simulink library "MEKF_ValidityTest_Lib2018"  (R2018b)
settings: Solver=VariableStepAuto  StartTime=0.0  StopTime=10.0  RelTol=1e-3
values from neighbouring files (symbols this model uses):
  Beta_init = Beta    [MEKF_ScriptandSimulink_Test.m]
  del_t = tspan(2)-tspan(1)    [MEKF_ScriptandSimulink_Test.m]
  P_sq_init = P_sq    [MEKF_ScriptandSimulink_Test.m]
  q = [q(:,2),q(:,3),q(:,4),q(:,1)]    [MEKF_ScriptandSimulink_Test.m]
  Q_sq = chol((gamma*Q_k*gamma'),'lower')    [MEKF_ScriptandSimulink_Test.m]
  qe_init = qe    [MEKF_ScriptandSimulink_Test.m]
  R_sq = chol(R,'lower')    [MEKF_ScriptandSimulink_Test.m]
libraries: MEKF_LibraryR2018b x13, aerolibutil x12, dspmtrx3 x7, sharedutil x6, $bdroot x2
(part 2 of 2)

== system MEKF_ValidityTest_Lib2018/MEKF with Validity Check/If All Sensors Valid/Kalman Gain ==
  P_sq : Inport
  q_est : Inport  Port=2
  SunVector_Inertial : Inport  Port=3
  "Mag_vec " : Inport  Port=4
  Constant : Constant  Value=R_sq  VectorParams1D=off
  Create H matrix : Subsystem
  Demux : Demux
  Divide : Product  Inputs=/  Multiplication=Matrix(*)
  MATLAB Function2 : MATLAB Function  TreatAsAtomicUnit=on
  Makes Xi(q) Matrix : Subsystem
  Matrix Concatenate : Concatenate  Mode=Multidimensional array
  Matrix Multiply1 : Product  Multiplication=Matrix(*)
  Mux : Mux
  Quaternion Rotation : aerolibutil/Quaternion Rotation
  Quaternion Rotation1 : aerolibutil/Quaternion Rotation
  P_square root plus : Outport
  Xi(q) : Outport  Port=2
  est_measurement : Outport  Port=3
  Kalman Gain K : Outport  Port=4
  wires:
  Divide/1 -> Matrix Multiply1/2
  MATLAB Function2/1(W) -> Matrix Multiply1/1
  Create H matrix/1(H) -> MATLAB Function2/3(H)  "Sensitivity Matrix"
  MATLAB Function2/2(sq_Bk) -> Divide/1
  P_sq/1 -> MATLAB Function2/2("P_sq ")
  Matrix Multiply1/1 -> Kalman Gain K/1  "Kalman Gain K"
  SunVector_Inertial/1 -> Quaternion Rotation/2
  Constant/1 -> MATLAB Function2/1(R_sq)
  MATLAB Function2/3(P_sq) -> P_square root plus/1  "P_square root plus"
  Demux/1 -> Mux/2
  Demux/2 -> Mux/3
  Demux/3 -> Mux/4
  Demux/4 -> Mux/1
  Makes Xi(q) Matrix/1(Xi(q)) -> Xi(q)/1
  q_est/1 -> [q_est]
  [q_est] -> Demux/1
  [q_est] -> Makes Xi(q) Matrix/1(qest)
  Quaternion Rotation/1 -> [rb_hat]  "product A(q)*R_i"
  [rb_hat] -> Create H matrix/1(rb_hat)
  "Mag_vec "/1 -> Quaternion Rotation1/2
  Quaternion Rotation1/1 -> [bhat]  "product A(q)*B_i"
  Mux/1 -> [qmix]
  [qmix] -> Quaternion Rotation1/1
  [qmix] -> Quaternion Rotation/1
  [bhat] -> Create H matrix/2(bb_hat)
  [rb_hat] -> Matrix Concatenate/1
  [bhat] -> Matrix Concatenate/2
  Matrix Concatenate/1 -> est_measurement/1

== system MEKF_ValidityTest_Lib2018/MEKF with Validity Check/If All Sensors Valid/MEASUREMENT UPDATE TO q AND COVARIANCE2 ==
  Xi_q : Inport
  r_est : Inport  Port=2
  Kalman Gain : Inport  Port=3
  q_est minus : Inport  Port=4
  Beta_est : Inport  Port=5
  Rb : Inport  Port=6
  Create Measurement Residual : Sum  Inputs=+-
  Demux : Demux  Outputs=2
  Normalize_q : Subsystem
  Product : Product  Inputs=**  Multiplication=Matrix(*)
  Product1 : Product  Multiplication=Matrix(*)
  Sum : Sum  Inputs=|++
  "Updating Beta Bias " : Sum  Inputs=|++
  gain1 : Gain  Gain=0.5
  Measurement updated q estimate : Outport
  Beta Updated : Outport  Port=2
  wires:
  Demux/1 -> Product/2  "Delta Alpha"
  gain1/1 -> Product/1  "0.5*Xi_q"
  Demux/2 -> "Updating Beta Bias "/1  "Delta Beta"
  Product/1 -> Sum/1
  Product1/1 -> Demux/1  "del_x"
  r_est/1 -> Create Measurement Residual/2
  Create Measurement Residual/1 -> Product1/2  "Measurement Residual"
  "Updating Beta Bias "/1 -> Beta Updated/1  "Beta Updated"
  Beta_est/1 -> "Updating Beta Bias "/2  "Beta_estimated"
  q_est minus/1 -> Sum/2
  Kalman Gain/1 -> Product1/1
  Rb/1 -> Create Measurement Residual/1
  Xi_q/1 -> gain1/1  "quaternion Propagation Matrix"
  Sum/1 -> Normalize_q/1(Estimated Quaternion)  "Estimated Quaternion"
  Normalize_q/1(q_normalized) -> Measurement updated q estimate/1

== system MEKF_ValidityTest_Lib2018/MEKF with Validity Check/If All Sensors Valid/TIME PROPAGATION of Q_EST, COVARIANCE ==
  P_square root plus : Inport
  qe : Inport  Port=2
  Updated bias : Inport  Port=3
  omega_meas : Inport  Port=4
  Constant{,1..3} (4 alike) : Constant  Value=del_t
  Constant11 : Constant  Value=0.5
  Constant13 : Constant  Value=Q_sq  VectorParams1D=off
  Gain : Gain  Gain=0.5
  MATLAB Function : MATLAB Function  TreatAsAtomicUnit=on
  MATLAB Function1 : MATLAB Function  TreatAsAtomicUnit=on
  MATLAB Function10 : MATLAB Function  TreatAsAtomicUnit=on
  MATLAB Function11 : MATLAB Function  TreatAsAtomicUnit=on
  MATLAB Function7 : MATLAB Function  TreatAsAtomicUnit=on
  MATLAB Function8 : MATLAB Function  TreatAsAtomicUnit=on
  MATLAB Function9 : MATLAB Function  TreatAsAtomicUnit=on
  Product : Product  Multiplication=Matrix(*)
  Psi : Subsystem
  cos_omega : Subsystem
  SqR P(k+1) : Outport
  qest(k+1) : Outport  Port=2
  Angular Velo Est : Outport  Port=3
  wires:
  Constant3/1 -> MATLAB Function8/4(del_t)
  MATLAB Function7/1(Psi_cross) -> MATLAB Function8/1(Psi_x)
  MATLAB Function11/1(P_sq) -> SqR P(k+1)/1  "C gets QR decomped to propagate sqrt(P)"
  MATLAB Function8/1(Omega_omega) -> Product/1  "q propagation matrix (nothing to do with angular velo)"
  MATLAB Function9/1(omega_cross_matrix) -> MATLAB Function10/4(omega_x)
  MATLAB Function10/1(State_Trans_matrix) -> MATLAB Function11/1(Phi_discrete)  "State Transition matrix to proagate P"
  Product/1 -> qest(k+1)/1  "Time Propagated q"
  Constant13/1 -> MATLAB Function11/2(Q_sq)  "process noise chol decomped covariance matrix"
  omega_meas/1 -> MATLAB Function1/2(mu)
  Updated bias/1 -> MATLAB Function1/1(nu)
  MATLAB Function/1(om_mag) -> [om_mag]  "om_mag"
  [om_mag] -> MATLAB Function10/3(om_mag)
  [om_mag] -> MATLAB Function8/3(om_mag)
  Constant1/1 -> MATLAB Function10/1(del_t)
  P_square root plus/1 -> [P_sq_plus]
  [P_sq_plus] -> MATLAB Function11/3("P_sq ")
  [omega_estj] -> MATLAB Function9/1(omega)
  [nonmergew] -> Angular Velo Est/1
  qe/1 -> [qe]
  [qe] -> Product/2
  [om_mag] -> cos_omega/1(In1)
  Constant/1 -> cos_omega/2(In2)
  [om_mag] -> cos_omega/3(In3)
  cos_omega/1(cos_omega) -> MATLAB Function10/2(cos_omega)  "cos_omega"
  Psi/1(Psi) -> MATLAB Function8/2(Psi), MATLAB Function7/1(Psi)  "Psi Matrix"
  Constant2/1 -> Psi/1(In1)
  Constant11/1 -> Psi/2(In2)
  [omega_estj] -> Psi/5(In4)
  [om_mag] -> Psi/3(In3), Psi/4(In5)
  MATLAB Function1/2(om_estbranch) -> Gain/1  "omega est"
  Gain/1 -> [omega_estj], MATLAB Function/1(omega_est)
  MATLAB Function1/1(om_est) -> [nonmergew]  "om_mag"

== system MEKF_ValidityTest_Lib2018/MEKF with Validity Check/If Gyros Valid, Sun or Mag Sensor Invlaid/Subsystem ==
  P_sq : Inport
  q_est1 : Inport  Port=2
  SunVector_Inertial : Inport  Port=3
  "Mag_vec " : Inport  Port=4
  Constant : Constant  Value=R_sq*100000000  VectorParams1D=off
  Create H matrix : MEKF_LibraryR2018b/Multiplicative Extended Kalman Filter/Kalman Gain/Create H matrix  SystemSampleTime=-1
  Demux : Demux
  Divide : Product  Inputs=/  Multiplication=Matrix(*)
  MATLAB Function2 : MEKF_LibraryR2018b/Multiplicative Extended Kalman Filter/Kalman Gain/MATLAB Function2  SystemSampleTime=-1
  Makes Xi(q) Matrix : MEKF_LibraryR2018b/Multiplicative Extended Kalman Filter/Kalman Gain/Makes Xi(q) Matrix  SystemSampleTime=-1
  Matrix Concatenate : Concatenate  Mode=Multidimensional array
  Matrix Multiply1 : Product  Multiplication=Matrix(*)
  Mux2 : Mux
  Quaternion Rotation2 : aerolibutil/Quaternion Rotation
  Quaternion Rotation3 : aerolibutil/Quaternion Rotation
  Xi(q) : Outport
  Kalman Gain K : Outport  Port=2
  P_square root plus : Outport  Port=3
  est_measurement : Outport  Port=4
  wires:
  Mux2/1 -> [qmix]
  q_est1/1 -> [q_est]
  P_sq/1 -> MATLAB Function2/2
  [q_est] -> Demux/1
  Demux/2 -> Mux2/3
  [q_est] -> Makes Xi(q) Matrix/1
  "Mag_vec "/1 -> Quaternion Rotation3/2
  Matrix Concatenate/1 -> est_measurement/1
  [bhat] -> Create H matrix/2
  Demux/1 -> Mux2/2
  [rb_hat] -> Matrix Concatenate/1
  Demux/4 -> Mux2/1
  [bhat] -> Matrix Concatenate/2
  [rb_hat] -> Create H matrix/1
  Quaternion Rotation2/1 -> [rb_hat]  "product A(q)*R_i"
  Quaternion Rotation3/1 -> [bhat]  "product A(q)*B_i"
  [qmix] -> Quaternion Rotation3/1
  Divide/1 -> Matrix Multiply1/2
  SunVector_Inertial/1 -> Quaternion Rotation2/2
  [qmix] -> Quaternion Rotation2/1
  Demux/3 -> Mux2/4
  Makes Xi(q) Matrix/1 -> Xi(q)/1
  MATLAB Function2/2 -> Divide/1
  Matrix Multiply1/1 -> Kalman Gain K/1  "Kalman Gain K"
  MATLAB Function2/3 -> P_square root plus/1  "P_square root plus"
  Create H matrix/1 -> MATLAB Function2/3  "Sensitivity Matrix"
  MATLAB Function2/1 -> Matrix Multiply1/1
  Constant/1 -> MATLAB Function2/1

== system MEKF_ValidityTest_Lib2018/MEKF with Validity Check/If Gyros Valid, Sun or Mag Sensor Invlaid/Subsystem1 ==
  Xi_q : Inport
  r_est : Inport  Port=2
  Kalman Gain : Inport  Port=3
  q_est minus : Inport  Port=4
  Beta_est : Inport  Port=5
  Rb : Inport  Port=6
  Create Measurement Residual : Sum  Inputs=+-
  Demux : Demux  Outputs=2
  Normalize_q : MEKF_LibraryR2018b/Multiplicative Extended Kalman Filter/MEASUREMENT UPDATE TO q AND COVARIANCE2/Normalize_q  SystemSampleTime=-1
  Product : Product  Inputs=**  Multiplication=Matrix(*)
  Product1 : Product  Multiplication=Matrix(*)
  Sum : Sum  Inputs=|++
  "Updating Beta Bias " : Sum  Inputs=|++
  gain1 : Gain  Gain=0.5
  Measurement updated q estimate : Outport
  Beta Updated : Outport  Port=2
  wires:
  Demux/2 -> "Updating Beta Bias "/1  "Delta Beta"
  Xi_q/1 -> gain1/1
  "Updating Beta Bias "/1 -> Beta Updated/1  "Beta Updated"
  Kalman Gain/1 -> Product1/1
  Create Measurement Residual/1 -> Product1/2  "Measurement Residual"
  Rb/1 -> Create Measurement Residual/1
  Demux/1 -> Product/2  "Delta Alpha"
  r_est/1 -> Create Measurement Residual/2
  Sum/1 -> Normalize_q/1  "Estimated Quaternion"
  Beta_est/1 -> "Updating Beta Bias "/2
  q_est minus/1 -> Sum/2
  Normalize_q/1 -> Measurement updated q estimate/1
  gain1/1 -> Product/1  "0.5*Xi_q"
  Product/1 -> Sum/1
  Product1/1 -> Demux/1  "del_x"

== system MEKF_ValidityTest_Lib2018/MEKF with Validity Check/If Gyros Valid, Sun or Mag Sensor Invlaid/Subsystem2 ==
  Square Root Covariane at next Time step becomes sqrt Pk minus : Inport
  Matrix Multiply : Product  Multiplication=Matrix(*)
  Transpose : Math  Operator=transpose  SaturateOnIntegerOverflow=on
  Out1 : Outport
  wires:
  Matrix Multiply/1 -> Out1/1
  Transpose/1 -> Matrix Multiply/2
  Square Root Covariane at next Time step becomes sqrt Pk minus/1 -> Transpose/1, Matrix Multiply/1

== system MEKF_ValidityTest_Lib2018/MEKF with Validity Check/If Gyros Valid, Sun or Mag Sensor Invlaid/Subsystem3 ==
  P_square root plus : Inport
  qe : Inport  Port=2
  Updated bias : Inport  Port=3
  omega_meas : Inport  Port=4
  Constant10 : Constant  Value=del_t
  Constant11 : Constant  Value=0.5
  Constant13 : Constant  Value=Q_sq  VectorParams1D=off
  MATLAB Function : MEKF_LibraryR2018b/Multiplicative Extended Kalman Filter/TIME PROPAGATION of Q_EST, COVARIANCE/MATLAB Function  SystemSampleTime=-1
  MATLAB Function10 : MEKF_LibraryR2018b/Multiplicative Extended Kalman Filter/TIME PROPAGATION of Q_EST, COVARIANCE/MATLAB Function10  SystemSampleTime=-1
  MATLAB Function11 : MEKF_LibraryR2018b/Multiplicative Extended Kalman Filter/TIME PROPAGATION of Q_EST, COVARIANCE/MATLAB Function11  SystemSampleTime=-1
  MATLAB Function7 : MEKF_LibraryR2018b/Multiplicative Extended Kalman Filter/TIME PROPAGATION of Q_EST, COVARIANCE/MATLAB Function7  SystemSampleTime=-1
  MATLAB Function8 : MEKF_LibraryR2018b/Multiplicative Extended Kalman Filter/TIME PROPAGATION of Q_EST, COVARIANCE/MATLAB Function8  SystemSampleTime=-1
  MATLAB Function9 : MEKF_LibraryR2018b/Multiplicative Extended Kalman Filter/TIME PROPAGATION of Q_EST, COVARIANCE/MATLAB Function9  SystemSampleTime=-1
  Product : Product  Multiplication=Matrix(*)
  Psi : MEKF_LibraryR2018b/Multiplicative Extended Kalman Filter/TIME PROPAGATION of Q_EST, COVARIANCE/Psi  SystemSampleTime=-1
  cos_omega : MEKF_LibraryR2018b/Multiplicative Extended Kalman Filter/TIME PROPAGATION of Q_EST, COVARIANCE/cos_omega  SystemSampleTime=-1
  subtract bias from omega meas : Sum  Inputs=|-+
  SqR P(k+1) : Outport
  qest(k+1) : Outport  Port=2
  Angular Velo Est : Outport  Port=3
  wires:
  MATLAB Function/1 -> [om_mag]  "om_mag"
  Psi/1 -> MATLAB Function8/2, MATLAB Function7/1  "Psi Matrix"
  [om_mag] -> Psi/3, Psi/4
  Constant11/1 -> Psi/2
  [qe] -> Product/2
  [del_t] -> Psi/1
  [omega_est] -> Angular Velo Est/1
  [del_t] -> MATLAB Function10/1
  [om_mag] -> MATLAB Function8/3
  MATLAB Function8/1 -> Product/1  "q propagation matrix (nothing to do with angular velo)"
  MATLAB Function10/1 -> MATLAB Function11/1  "State Transition matrix to proagate P"
  [omega_est] -> Psi/5
  [omega_est] -> MATLAB Function9/1
  [om_mag] -> MATLAB Function10/3
  [del_t] -> MATLAB Function8/4
  [del_t] -> cos_omega/2
  [om_mag] -> cos_omega/3
  MATLAB Function11/1 -> SqR P(k+1)/1  "C gets QR decomped to propagate sqrt(P)"
  [P_sq_plus] -> MATLAB Function11/3
  qe/1 -> [qe]
  P_square root plus/1 -> [P_sq_plus]
  MATLAB Function9/1 -> MATLAB Function10/4
  cos_omega/1 -> MATLAB Function10/2  "cos_omega"
  omega_meas/1 -> subtract bias from omega meas/2
  subtract bias from omega meas/1 -> MATLAB Function/1, [omega_est]  "omega est"
  Product/1 -> qest(k+1)/1  "Time Propagated q"
  Updated bias/1 -> subtract bias from omega meas/1
  Constant10/1 -> [del_t]  "del_t"
  MATLAB Function7/1 -> MATLAB Function8/1
  [om_mag] -> cos_omega/1
  Constant13/1 -> MATLAB Function11/2  "process noise chol decomped covariance matrix"

== system MEKF_ValidityTest_Lib2018/MEKF (All Sensors INVALID)/Kalman Gain/Create H matrix/3x3 0 matrix ==
  Create 3x3 Matrix : sharedutil/Create 3x3 Matrix  aMode=aMode
  Zero : Constant  Value=0  OutDataTypeStr=Inherit: Inherit via back propagation
  0 3x3 : Outport
  wires:
  Create 3x3 Matrix/1 -> 0 3x3/1
  Zero/1 -> Create 3x3 Matrix/4, Create 3x3 Matrix/3, Create 3x3 Matrix/2, Create 3x3 Matrix/5, Create 3x3 Matrix/1, Create 3x3 Matrix/6, Create 3x3 Matrix/7, Create 3x3 Matrix/8, Create 3x3 Matrix/9

== system MEKF_ValidityTest_Lib2018/MEKF (Sun, Mag:VALID Sensors Gyro: INVALID Sensor)/Kalman Gain/Create H matrix/3x3 0 matrix ==
  Create 3x3 Matrix : sharedutil/Create 3x3 Matrix  aMode=aMode
  Zero : Constant  Value=0  OutDataTypeStr=Inherit: Inherit via back propagation
  0 3x3 : Outport
  wires:
  Zero/1 -> Create 3x3 Matrix/9, Create 3x3 Matrix/8, Create 3x3 Matrix/7, Create 3x3 Matrix/6, Create 3x3 Matrix/1, Create 3x3 Matrix/5, Create 3x3 Matrix/2, Create 3x3 Matrix/3, Create 3x3 Matrix/4
  Create 3x3 Matrix/1 -> 0 3x3/1

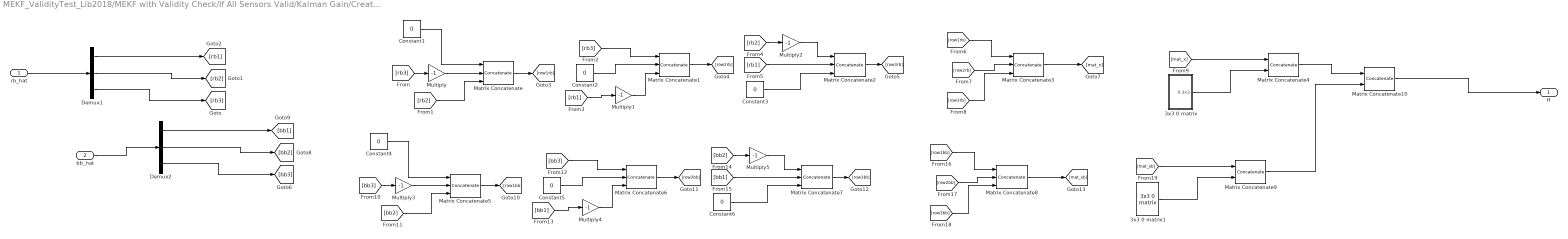
== system MEKF_ValidityTest_Lib2018/MEKF with Validity Check/If All Sensors Valid/Kalman Gain/Create H matrix ==
  rb_hat : Inport
  bb_hat : Inport  Port=2
  3x3 0 matrix : Subsystem
  3x3 0 matrix1 : MEKF_LibraryR2018b/Multiplicative Extended Kalman Filter/Kalman Gain/Create H matrix/3x3 0 matrix  SystemSampleTime=-1
  Constant{1..6} (6 alike) : Constant  Value=0
  Demux1 : Demux  Outputs=3
  Demux2 : Demux  Outputs=3
  Matrix Concatenate{,1..2,5..7} (6 alike) : Concatenate  NumInputs=3  Mode=Multidimensional array  ConcatenateDimension=2
  Matrix Concatenate10 : Concatenate  Mode=Multidimensional array
  Matrix Concatenate3 : Concatenate  NumInputs=3  Mode=Multidimensional array
  Matrix Concatenate4 : Concatenate  Mode=Multidimensional array  ConcatenateDimension=2
  Matrix Concatenate8 : Concatenate  NumInputs=3  Mode=Multidimensional array
  Matrix Concatenate9 : Concatenate  Mode=Multidimensional array  ConcatenateDimension=2
  Multiply{,1..5} (6 alike) : Gain  Gain=-1
  H : Outport
  wires:
  Matrix Concatenate1/1 -> [row2rb]
  Multiply/1 -> Matrix Concatenate/2
  [mat_x] -> Matrix Concatenate4/1
  Demux1/2 -> [rb2]
  Multiply2/1 -> Matrix Concatenate2/1
  [row3rb] -> Matrix Concatenate3/3
  Matrix Concatenate/1 -> [row1rb]
  Matrix Concatenate2/1 -> [row3rb]
  [rb1] -> Multiply1/1
  [rb3] -> Multiply/1
  Multiply1/1 -> Matrix Concatenate1/3
  Constant3/1 -> Matrix Concatenate2/3
  3x3 0 matrix/1(0 3x3) -> Matrix Concatenate4/2
  [rb2] -> Multiply2/1
  [rb2] -> Matrix Concatenate/3
  [rb3] -> Matrix Concatenate1/1
  [row2rb] -> Matrix Concatenate3/2
  Constant1/1 -> Matrix Concatenate/1
  [row1rb] -> Matrix Concatenate3/1
  Demux1/1 -> [rb1]
  Matrix Concatenate3/1 -> [mat_x]
  Constant2/1 -> Matrix Concatenate1/2
  [rb1] -> Matrix Concatenate2/2
  Demux1/3 -> [rb3]
  rb_hat/1 -> Demux1/1
  Demux2/3 -> [bb3]
  bb_hat/1 -> Demux2/1
  Demux2/1 -> [bb1]
  Demux2/2 -> [bb2]
  Multiply5/1 -> Matrix Concatenate7/1
  [bb1] -> Matrix Concatenate7/2
  Constant4/1 -> Matrix Concatenate5/1
  Multiply3/1 -> Matrix Concatenate5/2
  Constant5/1 -> Matrix Concatenate6/2
  Multiply4/1 -> Matrix Concatenate6/3
  Matrix Concatenate5/1 -> [row1bb]
  [bb1] -> Multiply4/1
  Matrix Concatenate7/1 -> [row3bb]
  Constant6/1 -> Matrix Concatenate7/3
  [bb2] -> Matrix Concatenate5/3
  [bb3] -> Multiply3/1
  [bb3] -> Matrix Concatenate6/1
  [bb2] -> Multiply5/1
  Matrix Concatenate6/1 -> [row2bb]
  [row1bb] -> Matrix Concatenate8/1
  Matrix Concatenate8/1 -> [mat_xb]
  [row2bb] -> Matrix Concatenate8/2
  [row3bb] -> Matrix Concatenate8/3
  3x3 0 matrix1/1 -> Matrix Concatenate9/2
  Matrix Concatenate9/1 -> Matrix Concatenate10/2
  [mat_xb] -> Matrix Concatenate9/1
  Matrix Concatenate4/1 -> Matrix Concatenate10/1
  Matrix Concatenate10/1 -> H/1

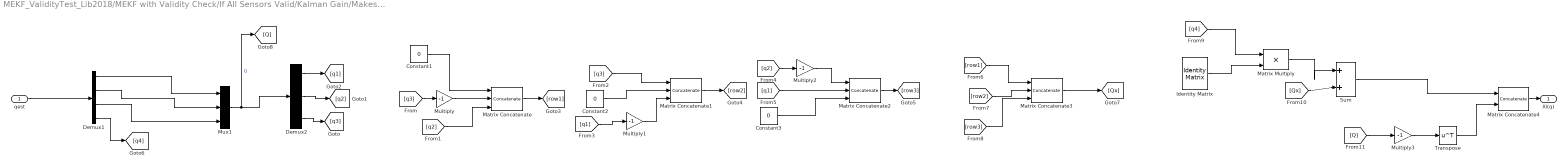
== system MEKF_ValidityTest_Lib2018/MEKF with Validity Check/If All Sensors Valid/Kalman Gain/Makes Xi(q) Matrix ==
  qest : Inport
  Constant1 : Constant  Value=0
  Constant2 : Constant  Value=0
  Constant3 : Constant  Value=0
  Demux1 : Demux
  Demux2 : Demux  Outputs=3
  Identity Matrix : dspmtrx3/Identity Matrix  Inherit=off  N=3  Ts=1  dataType=double  isSigned=on  wordLen=16  udDataType=sfix(16)  fracBitsMode=Best precision  numFracBits=15  OutDataTypeStr=double  LastOutDataTypeStr=double
      settings: SourceProductName=DSP System Toolbox
  Matrix Concatenate : Concatenate  NumInputs=3  Mode=Multidimensional array  ConcatenateDimension=2
  Matrix Concatenate1 : Concatenate  NumInputs=3  Mode=Multidimensional array  ConcatenateDimension=2
  Matrix Concatenate2 : Concatenate  NumInputs=3  Mode=Multidimensional array  ConcatenateDimension=2
  Matrix Concatenate3 : Concatenate  NumInputs=3  Mode=Multidimensional array
  Matrix Concatenate4 : Concatenate  Mode=Multidimensional array
  Matrix Multiply : Product  Inputs=**
  Multiply{,1..3} (4 alike) : Gain  Gain=-1
  Mux1 : Mux  Inputs=3
  Sum : Sum  Inputs=|++
  Transpose : Math  Operator=transpose  SaturateOnIntegerOverflow=on
  Xi(q) : Outport
  wires:
  Multiply2/1 -> Matrix Concatenate2/1
  [q1] -> Matrix Concatenate2/2
  Matrix Multiply/1 -> Sum/1
  Matrix Concatenate1/1 -> [row2]
  Constant1/1 -> Matrix Concatenate/1
  Matrix Concatenate3/1 -> [Qx]
  [q2] -> Matrix Concatenate/3
  Mux1/1 -> Demux2/1, [Q]  "Q"
  Constant2/1 -> Matrix Concatenate1/2
  Demux1/2 -> Mux1/2
  [row3] -> Matrix Concatenate3/3
  qest/1 -> Demux1/1
  Multiply3/1 -> Transpose/1
  [q4] -> Matrix Multiply/1
  [q3] -> Matrix Concatenate1/1
  Demux2/2 -> [q2]
  Sum/1 -> Matrix Concatenate4/1
  [q2] -> Multiply2/1
  Demux1/4 -> [q4]
  [row2] -> Matrix Concatenate3/2
  Demux1/1 -> Mux1/1
  Demux1/3 -> Mux1/3
  Matrix Concatenate2/1 -> [row3]
  [Qx] -> Sum/2
  Multiply/1 -> Matrix Concatenate/2
  [row1] -> Matrix Concatenate3/1
  [Q] -> Multiply3/1
  Demux2/1 -> [q1]
  Transpose/1 -> Matrix Concatenate4/2
  Identity Matrix/1 -> Matrix Multiply/2
  [q3] -> Multiply/1
  Matrix Concatenate/1 -> [row1]
  Demux2/3 -> [q3]
  Constant3/1 -> Matrix Concatenate2/3
  [q1] -> Multiply1/1
  Multiply1/1 -> Matrix Concatenate1/3
  Matrix Concatenate4/1 -> Xi(q)/1

== system MEKF_ValidityTest_Lib2018/MEKF with Validity Check/If All Sensors Valid/MEASUREMENT UPDATE TO q AND COVARIANCE2/Normalize_q ==
  note: Rearrange_Quat
  note: Rearrange_Quat_back
  Estimated Quaternion : Inport
  Demux : Demux
  Demux1 : Demux
  Mux : Mux
  Mux1 : Mux
  Quaternion Normalize : sharedutil/Quaternion Normalize  aMode=aMode
      settings: SourceProductName=Aerospace Blockset  SourceProductBaseCode=AE
  q_normalized : Outport
  wires:
  Mux1/1 -> Quaternion Normalize/1
  Demux1/4 -> Mux1/1
  Demux/4 -> Mux/3
  Demux/3 -> Mux/2
  Demux/2 -> Mux/1
  Demux1/3 -> Mux1/4
  Mux/1 -> q_normalized/1
  Demux1/1 -> Mux1/2
  Demux1/2 -> Mux1/3
  Demux/1 -> Mux/4
  Quaternion Normalize/1 -> Demux/1  "Measurement updated q estimate"
  Estimated Quaternion/1 -> Demux1/1

== system MEKF_ValidityTest_Lib2018/MEKF with Validity Check/If All Sensors Valid/TIME PROPAGATION of Q_EST, COVARIANCE/Psi ==
  In1 : Inport
  In2 : Inport  Port=2
  In3 : Inport  Port=3
  In5 : Inport  Port=4
  In4 : Inport  Port=5
  Divide : Product  Inputs=***
  Divide1 : Product  Inputs=**/
  Sin : Trigonometry
  Psi : Outport
  wires:
  In1/1 -> Divide/1
  Divide/1 -> Sin/1  "om_mag times0.5*del_t"
  In5/1 -> Divide1/3
  In4/1 -> Divide1/2
  Divide1/1 -> Psi/1  "Psi"
  In3/1 -> Divide/3
  Sin/1 -> Divide1/1  "sin(om_mag*0.5*del_t)"
  In2/1 -> Divide/2

== system MEKF_ValidityTest_Lib2018/MEKF with Validity Check/If All Sensors Valid/TIME PROPAGATION of Q_EST, COVARIANCE/cos_omega ==
  In1 : Inport
  In2 : Inport  Port=2
  In3 : Inport  Port=3
  Constant12 : Constant
  Cos : Trigonometry  Operator=cos
  Divide2 : Product  Inputs=**
  Divide3 : Product  Inputs=*/
  Square : Math  Operator=square  SaturateOnIntegerOverflow=on
  Sum3 : Sum  Inputs=|+-
  cos_omega : Outport
  wires:
  Divide2/1 -> Cos/1
  In3/1 -> Square/1
  Divide3/1 -> cos_omega/1  "cos_omega"
  Constant12/1 -> Sum3/1
  Square/1 -> Divide3/2  "omega mag squared"
  In1/1 -> Divide2/1
  Cos/1 -> Sum3/2
  In2/1 -> Divide2/2
  Sum3/1 -> Divide3/1  "(1-cos(om_mag*del_t))"

== system MEKF_ValidityTest_Lib2018/MEKF with Validity Check/If All Sensors Valid/Kalman Gain/Create H matrix/3x3 0 matrix ==
  Create 3x3 Matrix : sharedutil/Create 3x3 Matrix  aMode=aMode
  Zero : Constant  Value=0  OutDataTypeStr=Inherit: Inherit via back propagation
  0 3x3 : Outport
  wires:
  Zero/1 -> Create 3x3 Matrix/9, Create 3x3 Matrix/8, Create 3x3 Matrix/7, Create 3x3 Matrix/6, Create 3x3 Matrix/1, Create 3x3 Matrix/5, Create 3x3 Matrix/2, Create 3x3 Matrix/3, Create 3x3 Matrix/4
  Create 3x3 Matrix/1 -> 0 3x3/1

== matlab function MEKF_ValidityTest_Lib2018/MEKF with Validity Check/If All Sensors Valid/Kalman Gain/MATLAB Function2 ==
  data: R_sq input; W output; P_sq input; H input; sq_Bk output; P_sq output
function [W,sq_Bk,P_sq] = fcnAQR(R_sq,P_sq,H)
%#codegen
[nr,mr] = size(R_sq);
[np,mp] = size(P_sq);
A_QR = [R_sq',zeros(nr,np);(P_sq')*H', P_sq'];

[TA,UA] = qr(A_QR);
        P_sq = UA(7:12,7:12)'; %Updated P_sq
        W = UA(1:6,7:12)';
%        
        sq_Bk = UA(1:6,1:6)';

== matlab function MEKF_ValidityTest_Lib2018/MEKF with Validity Check/If All Sensors Valid/TIME PROPAGATION of Q_EST, COVARIANCE/MATLAB Function1 ==
  data: nu input; om_est output; mu input; om_estbranch output
function [om_est,om_estbranch] = om2_est(nu,mu)

om_est = mu-nu;
om_estbranch =2*( mu-nu);

== matlab function MEKF_ValidityTest_Lib2018/MEKF with Validity Check/If All Sensors Valid/TIME PROPAGATION of Q_EST, COVARIANCE/MATLAB Function7 ==
  data: Psi input; Psi_cross output
function Psi_cross = Psi_cross_matrix(Psi)
%#codegen

Psi_cross = [0 -Psi(3) Psi(2);Psi(3) 0 -Psi(1);-Psi(2) Psi(1) 0];

== matlab function MEKF_ValidityTest_Lib2018/MEKF with Validity Check/If All Sensors Valid/TIME PROPAGATION of Q_EST, COVARIANCE/MATLAB Function8 ==
  data: Psi_x input; Psi input; om_mag input; del_t input; Omega_omega output
function Omega_omega = omega_omega_matrix(Psi_x,Psi,om_mag,del_t)
%#codegen

 Omega_omega = [(cos(0.5*om_mag*del_t)*eye(3) - Psi_x), Psi; -Psi', cos(0.5*om_mag*del_t)];

== matlab function MEKF_ValidityTest_Lib2018/MEKF with Validity Check/If All Sensors Valid/TIME PROPAGATION of Q_EST, COVARIANCE/MATLAB Function9 ==
  data: omega input; omega_cross_matrix output
function omega_cross_matrix = makes_omega_cross_matrix(omega)

omega_cross_matrix = [0 -omega(3) omega(2);omega(3) 0 -omega(1);-omega(2) omega(1) 0];

== matlab function MEKF_ValidityTest_Lib2018/MEKF with Validity Check/If All Sensors Valid/TIME PROPAGATION of Q_EST, COVARIANCE/MATLAB Function10 ==
  data: del_t input; cos_omega input; om_mag input; omega_x input; State_Trans_matrix output
function State_Trans_matrix = Phi_disc(del_t,cos_omega,om_mag,omega_x)
%#codegen

State_Trans_matrix = [(eye(3)-omega_x*sin(om_mag*del_t)/om_mag + (omega_x^2)*cos_omega),omega_x*cos_omega-eye(3)*del_t-omega_x^2*(om_mag*del_t-sin(om_mag*del_t))/om_mag^3;
            zeros(3,3),eye(3)];

== matlab function MEKF_ValidityTest_Lib2018/MEKF with Validity Check/If All Sensors Valid/TIME PROPAGATION of Q_EST, COVARIANCE/MATLAB Function11 ==
  data: Phi_discrete input; P_sq output; Q_sq input; P_sq input
function P_sq  = Cqr(Phi_discrete,Q_sq,P_sq)
%#codegen

C = [P_sq'*Phi_discrete';Q_sq'];
          [Tc,Uc] = qr(C);
%           Uc = full(Uc);
          sq_P_kp1 = Uc(1:6,1:6)';
%           P = sq_P_kp1'*sq_P_kp1;
          P_sq = sq_P_kp1;

== matlab function MEKF_ValidityTest_Lib2018/MEKF with Validity Check/If All Sensors Valid/TIME PROPAGATION of Q_EST, COVARIANCE/MATLAB Function ==
  data: omega_est input; om_mag output
function om_mag = om2_norm(omega_est)

om_mag = norm(omega_est);

== matlab function MEKF_ValidityTest_Lib2018/MEKF (Sun, Mag:VALID Sensors Gyro: INVALID Sensor)/Kalman Gain/MATLAB Function2 ==
  data: R_sq input; W output; P_sq input; H input; sq_Bk output; P_sq output
function [W,sq_Bk,P_sq] = fcnAQR(R_sq,P_sq,H)
%#codegen
[nr,mr] = size(R_sq);
[np,mp] = size(P_sq);
A_QR = [R_sq',zeros(nr,np);(P_sq')*H', P_sq'];

[TA,UA] = qr(A_QR);
        P_sq = UA(7:12,7:12)'; %Updated P_sq
        W = UA(1:6,7:12)';
%        
        sq_Bk = UA(1:6,1:6)';

== matlab function MEKF_ValidityTest_Lib2018/MEKF (Sun, Mag:VALID Sensors Gyro: INVALID Sensor)/Kalman Gain/MATLAB Function3 ==
  data: q_est input; Xi_q output
function Xi_q  = Xi_Phi_matrices(q_est)
%#codegen
        Q = [q_est(1:3,1)]; %change these q's to be q(1,1)
        Qx = [0 -q_est(3) q_est(2);q_est(3) 0 -q_est(1);-q_est(2) q_est(1) 0]; %cross product matrix of q
        Xi_q = [q_est(4)*eye(3)+Qx;-Q'];
%         Phi_q = [q_est(4)*eye(3)-Qx;-Q'];

== matlab function MEKF_ValidityTest_Lib2018/MEKF (Sun, Mag:VALID Sensors Gyro: INVALID Sensor)/Kalman Gain/MATLAB Function4 ==
  data: mat input; H output
function H = H_Matrix(mat)
%#codegen
mat_x = [0 -mat(3) mat(2);mat(3) 0 -mat(1);-mat(2) mat(1) 0];
H = [mat_x, zeros(3,3)];

== matlab function MEKF_ValidityTest_Lib2018/MEKF (Sun, Mag:VALID Sensors Gyro: INVALID Sensor)/TIME PROPAGATION of Q_EST, COVARIANCE/MATLAB Function ==
  data: omega_est input; om_mag output
function om_mag = om2_norm(omega_est)

om_mag = norm(omega_est);

== matlab function MEKF_ValidityTest_Lib2018/MEKF (Sun, Mag:VALID Sensors Gyro: INVALID Sensor)/TIME PROPAGATION of Q_EST, COVARIANCE/MATLAB Function10 ==
  data: del_t input; cos_omega input; om_mag input; omega_x input; State_Trans_matrix output
function State_Trans_matrix = Phi_disc(del_t,cos_omega,om_mag,omega_x)
%#codegen

State_Trans_matrix = [(eye(3)-omega_x*sin(om_mag*del_t)/om_mag + (omega_x^2)*cos_omega),omega_x*cos_omega-eye(3)*del_t-omega_x^2*(om_mag*del_t-sin(om_mag*del_t))/om_mag^3;
            zeros(3,3),eye(3)];

== matlab function MEKF_ValidityTest_Lib2018/MEKF (Sun, Mag:VALID Sensors Gyro: INVALID Sensor)/TIME PROPAGATION of Q_EST, COVARIANCE/MATLAB Function11 ==
  data: Phi_discrete input; P_sq output; Q_sq input; P_sq input
function P_sq  = Cqr(Phi_discrete,Q_sq,P_sq)
%#codegen

C = [P_sq'*Phi_discrete';Q_sq'];
          [Tc,Uc] = qr(C);
%           Uc = full(Uc);
          sq_P_kp1 = Uc(1:6,1:6)';
%           P = sq_P_kp1'*sq_P_kp1;
          P_sq = sq_P_kp1;

== matlab function MEKF_ValidityTest_Lib2018/MEKF (Sun, Mag:VALID Sensors Gyro: INVALID Sensor)/TIME PROPAGATION of Q_EST, COVARIANCE/MATLAB Function7 ==
  data: Psi input; Psi_cross output
function Psi_cross = Psi_cross_matrix(Psi)
%#codegen

Psi_cross = [0 -Psi(3) Psi(2);Psi(3) 0 -Psi(1);-Psi(2) Psi(1) 0];

== matlab function MEKF_ValidityTest_Lib2018/MEKF (Sun, Mag:VALID Sensors Gyro: INVALID Sensor)/TIME PROPAGATION of Q_EST, COVARIANCE/MATLAB Function8 ==
  data: Psi_x input; Psi input; om_mag input; del_t input; Omega_omega output
function Omega_omega = omega_omega_matrix(Psi_x,Psi,om_mag,del_t)
%#codegen

 Omega_omega = [(cos(0.5*om_mag*del_t)*eye(3) - Psi_x), Psi; -Psi', cos(0.5*om_mag*del_t)];

== matlab function MEKF_ValidityTest_Lib2018/MEKF (Sun, Mag:VALID Sensors Gyro: INVALID Sensor)/TIME PROPAGATION of Q_EST, COVARIANCE/MATLAB Function9 ==
  data: omega input; omega_cross_matrix output
function omega_cross_matrix = makes_omega_cross_matrix(omega)

omega_cross_matrix = [0 -omega(3) omega(2);omega(3) 0 -omega(1);-omega(2) omega(1) 0];

== matlab function MEKF_ValidityTest_Lib2018/MEKF (All Sensors INVALID)/Kalman Gain/MATLAB Function2 ==
  data: R_sq input; W output; P_sq input; H input; sq_Bk output; P_sq output
function [W,sq_Bk,P_sq] = fcnAQR(R_sq,P_sq,H)
%#codegen
[nr,mr] = size(R_sq);
[np,mp] = size(P_sq);
A_QR = [R_sq',zeros(nr,np);(P_sq')*H', P_sq'];

[TA,UA] = qr(A_QR);
        P_sq = UA(7:12,7:12)'; %Updated P_sq
        W = UA(1:6,7:12)';
%        
        sq_Bk = UA(1:6,1:6)';

== matlab function MEKF_ValidityTest_Lib2018/MEKF (All Sensors INVALID)/Kalman Gain/MATLAB Function3 ==
  data: q_est input; Xi_q output
function Xi_q  = Xi_Phi_matrices(q_est)
%#codegen
        Q = [q_est(1:3,1)]; %change these q's to be q(1,1)
        Qx = [0 -q_est(3) q_est(2);q_est(3) 0 -q_est(1);-q_est(2) q_est(1) 0]; %cross product matrix of q
        Xi_q = [q_est(4)*eye(3)+Qx;-Q'];
%         Phi_q = [q_est(4)*eye(3)-Qx;-Q'];

== matlab function MEKF_ValidityTest_Lib2018/MEKF (All Sensors INVALID)/Kalman Gain/MATLAB Function4 ==
  data: mat input; H output
function H = H_Matrix(mat)
%#codegen
mat_x = [0 -mat(3) mat(2);mat(3) 0 -mat(1);-mat(2) mat(1) 0];
H = [mat_x, zeros(3,3)];

== matlab function MEKF_ValidityTest_Lib2018/MEKF (All Sensors INVALID)/TIME PROPAGATION of Q_EST, COVARIANCE/MATLAB Function ==
  data: omega_est input; om_mag output
function om_mag = om2_norm(omega_est)

om_mag = norm(omega_est);

== matlab function MEKF_ValidityTest_Lib2018/MEKF (All Sensors INVALID)/TIME PROPAGATION of Q_EST, COVARIANCE/MATLAB Function10 ==
  data: del_t input; cos_omega input; om_mag input; omega_x input; State_Trans_matrix output
function State_Trans_matrix = Phi_disc(del_t,cos_omega,om_mag,omega_x)
%#codegen

State_Trans_matrix = [(eye(3)-omega_x*sin(om_mag*del_t)/om_mag + (omega_x^2)*cos_omega),omega_x*cos_omega-eye(3)*del_t-omega_x^2*(om_mag*del_t-sin(om_mag*del_t))/om_mag^3;
            zeros(3,3),eye(3)];

== matlab function MEKF_ValidityTest_Lib2018/MEKF (All Sensors INVALID)/TIME PROPAGATION of Q_EST, COVARIANCE/MATLAB Function11 ==
  data: Phi_discrete input; P_sq output; Q_sq input; P_sq input
function P_sq  = Cqr(Phi_discrete,Q_sq,P_sq)
%#codegen

C = [P_sq'*Phi_discrete';Q_sq'];
          [Tc,Uc] = qr(C);
%           Uc = full(Uc);
          sq_P_kp1 = Uc(1:6,1:6)';
%           P = sq_P_kp1'*sq_P_kp1;
          P_sq = sq_P_kp1;

== matlab function MEKF_ValidityTest_Lib2018/MEKF (All Sensors INVALID)/TIME PROPAGATION of Q_EST, COVARIANCE/MATLAB Function7 ==
  data: Psi input; Psi_cross output
function Psi_cross = Psi_cross_matrix(Psi)
%#codegen

Psi_cross = [0 -Psi(3) Psi(2);Psi(3) 0 -Psi(1);-Psi(2) Psi(1) 0];

== matlab function MEKF_ValidityTest_Lib2018/MEKF (All Sensors INVALID)/TIME PROPAGATION of Q_EST, COVARIANCE/MATLAB Function8 ==
  data: Psi_x input; Psi input; om_mag input; del_t input; Omega_omega output
function Omega_omega = omega_omega_matrix(Psi_x,Psi,om_mag,del_t)
%#codegen

 Omega_omega = [(cos(0.5*om_mag*del_t)*eye(3) - Psi_x), Psi; -Psi', cos(0.5*om_mag*del_t)];

== matlab function MEKF_ValidityTest_Lib2018/MEKF (All Sensors INVALID)/TIME PROPAGATION of Q_EST, COVARIANCE/MATLAB Function9 ==
  data: omega input; omega_cross_matrix output
function omega_cross_matrix = makes_omega_cross_matrix(omega)

omega_cross_matrix = [0 -omega(3) omega(2);omega(3) 0 -omega(1);-omega(2) omega(1) 0];
